simulink model "Simscape_Valve_Cylinder_4"  (R2014a)
settings: Solver=ode45  StartTime=0.0  StopTime=10.0  RelTol=1e-3
undefined symbols (not defined in the file): leakage_area
libraries: fl_lib x6
Description:
  | Copyright 2014 The MathWorks, Inc.
settings Model: Creator=smiller  LastModifiedBy=smiller
settings DataIOCC: SignalLoggingSaveFormat=ModelDataLogs
settings OptimizationCC: ExpressionDepthLimit=2147483647  InitFltsAndDblsToZero=on
settings DebuggingCC: SaveWithParameterizedLinksMsg=none  UnderspecifiedInitializationDetection=Classic  FcnCallInpInsideContextMsg=UseLocalSettings  StateNameClashWarn=warning
settings GRTTargetCC: TargetFcnLib=ansi_tfl_tmw.mat  CombineOutputUpdateFcns=off  GRTInterface=on

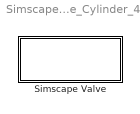
== system Simscape_Valve_Cylinder_4 ==
  Simscape Valve : Subsystem

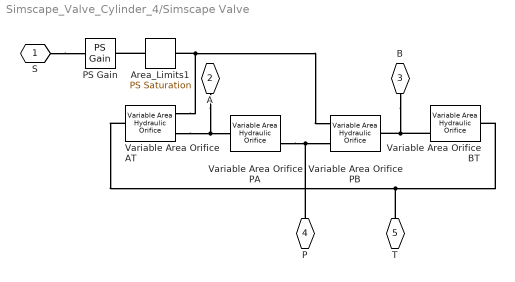
== system Simscape_Valve_Cylinder_4/Simscape Valve ==
  Area_Limits1 : fl_lib/Physical Signals/Nonlinear Operators/PS Saturation  upper_limit=1e-5 + leakage_area  lower_limit=leakage_area
  PS Gain : fl_lib/Physical Signals/Functions/PS Gain  gain=-1
  Variable Area Orifice AT : fl_lib/Hydraulic/Hydraulic Elements/Variable Area Hydraulic Orifice  C_d=0.7  Re_cr=12  min_area=1e-12 m^2  q_specify=off  q_priority=High  q=1 m^3/s  p_specify=off  p_priority=High  p=0 Pa
  Variable Area Orifice BT : fl_lib/Hydraulic/Hydraulic Elements/Variable Area Hydraulic Orifice  C_d=0.7  Re_cr=12  min_area=1e-12 m^2  q_specify=off  q_priority=High  q=1 m^3/s  p_specify=off  p_priority=High  p=0 Pa
  Variable Area Orifice PA : fl_lib/Hydraulic/Hydraulic Elements/Variable Area Hydraulic Orifice  C_d=0.7  Re_cr=12  min_area=1e-12 m^2  q_specify=off  q_priority=High  q=1 m^3/s  p_specify=off  p_priority=High  p=0 Pa
  Variable Area Orifice PB : fl_lib/Hydraulic/Hydraulic Elements/Variable Area Hydraulic Orifice  C_d=0.7  Re_cr=12  min_area=1e-12 m^2  q_specify=off  q_priority=High  q=1 m^3/s  p_specify=off  p_priority=High  p=0 Pa
  S : PMIOPort  Tag=PMCPort  Port=1  Side=Left
  A : PMIOPort  Tag=PMCPort  Port=2  Side=Right
  B : PMIOPort  Tag=PMCPort  Port=3  Side=Right
  P : PMIOPort  Tag=PMCPort  Port=4  Side=Left
  T : PMIOPort  Tag=PMCPort  Port=5  Side=Left
  connections:
  P/RConn1 -- Variable Area Orifice PA/LConn2 -- Variable Area Orifice PB/LConn2
  B/RConn1 -- Variable Area Orifice BT/LConn2 -- Variable Area Orifice PB/RConn1
  A/RConn1 -- Variable Area Orifice AT/LConn2 -- Variable Area Orifice PA/RConn1
  Variable Area Orifice AT/RConn1 -- T/RConn1 -- Variable Area Orifice BT/RConn1
  S/RConn1 -- PS Gain/LConn1
  Variable Area Orifice PB/LConn1 -- Variable Area Orifice AT/LConn1 -- Area_Limits1/RConn1
  Area_Limits1/LConn1 -- PS Gain/RConn1
